simulink model "counter7_0_5__5"  (R2018a)
settings: Solver=VariableStepAuto  StartTime=0.0  StopTime=10.0  RelTol=1e-3
settings Model: Creator=SONY  LastModifiedBy=SONY

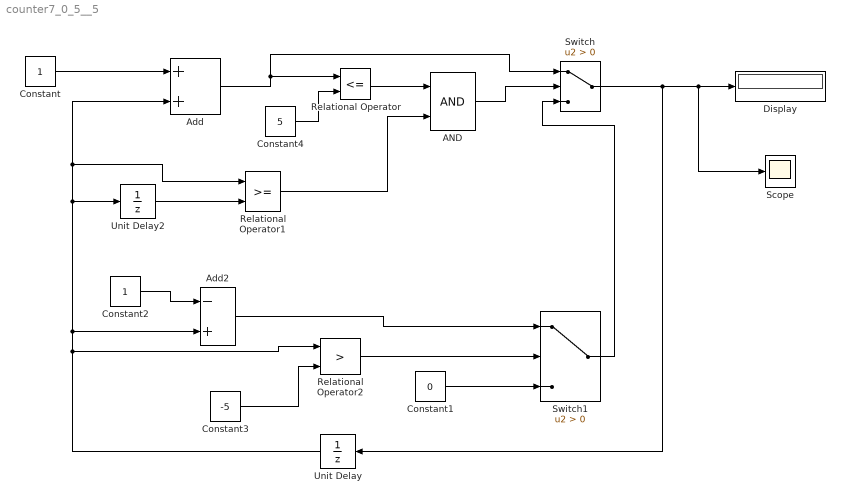
== system counter7_0_5__5 ==
  AND : Logic  AllPortsSameDT=off  OutDataTypeStr=boolean
  Add : Sum
  Add2 : Sum  Inputs=-+
  Constant : Constant
  Constant1 : Constant  Value=0
  Constant2 : Constant
  Constant3 : Constant  Value=-5
  Constant4 : Constant  Value=5
  Display : Display
  Relational Operator : RelationalOperator  Operator=<=  OutDataTypeStr=boolean  RndMeth=Simplest
  Relational Operator1 : RelationalOperator  OutDataTypeStr=boolean  RndMeth=Simplest
  Relational Operator2 : RelationalOperator  Operator=>  OutDataTypeStr=boolean  RndMeth=Simplest
  Scope : Scope
  Switch : Switch  Criteria=u2 > Threshold
  Switch1 : Switch  Criteria=u2 > Threshold
  Unit Delay : UnitDelay  InitialCondition=-1  SampleTime=-1
  Unit Delay2 : UnitDelay  InitialCondition=-2  SampleTime=-1
  wires:
  Relational Operator2/1 -> Switch1/2
  Unit Delay2/1 -> Relational Operator1/2
  Unit Delay/1 -> Relational Operator2/1, Unit Delay2/1, Relational Operator1/1, Add/2, Add2/2
  Constant4/1 -> Relational Operator/2
  Add2/1 -> Switch1/1
  Relational Operator/1 -> AND/1
  Switch1/1 -> Switch/3
  Switch/1 -> Unit Delay/1, Scope/1, Display/1
  Constant1/1 -> Switch1/3
  Constant/1 -> Add/1
  Relational Operator1/1 -> AND/2
  Constant3/1 -> Relational Operator2/2
  Constant2/1 -> Add2/1
  Add/1 -> Switch/1, Relational Operator/1
  AND/1 -> Switch/2
